simulink model "Panel_Equation"  (R2022b)
settings: Solver=VariableStepAuto  StartTime=0.0  StopTime=10.0  RelTol=1e-3
model workspace (MAT data in the model file):
  J = 8.6
  Kd = 5
settings Model: Creator=adlercohen  LastModifiedBy=adlercohen

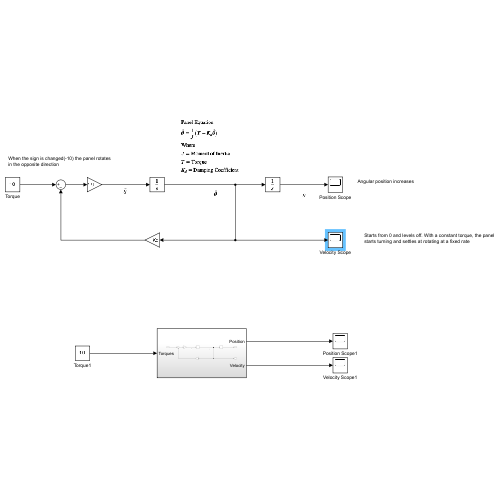
[thumbnail: Simulink's stored preview of the top-level diagram]
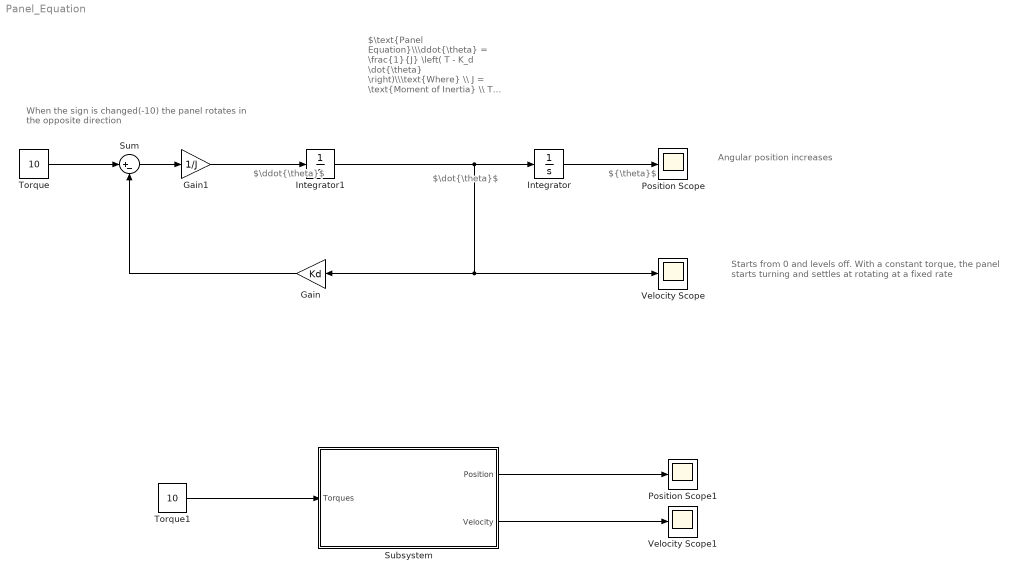
== system Panel_Equation ==
  note: When the sign is changed(-10) the panel rotates
      | in the opposite direction
  note: Starts from 0 and levels off. With a constant torque, the panel
      | starts turning and settles at rotating at a fixed rate
  note: Angular position increases
  note: $\dot{\theta}$
  note: $\text{Panel Equation}\\\ddot{\theta} = \frac{1}{J} \left( T - K_d \dot{\theta} \right)\\\text{Where} \\ J = \text{Moment of Inertia} \\ T = \text{Torque} \\ K_d = \text{Damping Coefficient}$
  note: $\ddot{\theta}$
  note: ${\theta}$
  Gain : Gain  Gain=Kd
  Gain1 : Gain  Gain=1/J
  Integrator : Integrator
  Integrator1 : Integrator
  Position Scope : Scope
  Position Scope1 : Scope
  Subsystem : Subsystem
  Sum : Sum  Inputs=|+-
  Torque : Constant  Value=10
  Torque1 : Constant  Value=10
  Velocity Scope : Scope
  Velocity Scope1 : Scope
  wires:
  Integrator1/1 -> Gain/1, Velocity Scope/1, Integrator/1
  Integrator/1 -> Position Scope/1
  Sum/1 -> Gain1/1
  Torque/1 -> Sum/1
  Gain/1 -> Sum/2
  Gain1/1 -> Integrator1/1
  Torque1/1 -> Subsystem/1(Torques)
  Subsystem/1(Position) -> Position Scope1/1
  Subsystem/2(Velocity) -> Velocity Scope1/1

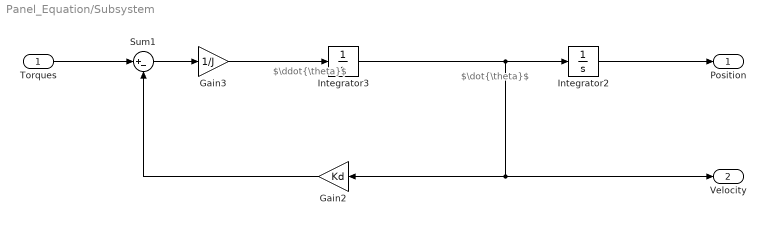
== system Panel_Equation/Subsystem ==
  note: $\ddot{\theta}$
  note: $\dot{\theta}$
  Torques : Inport
  Gain2 : Gain  Gain=Kd
  Gain3 : Gain  Gain=1/J
  Integrator2 : Integrator
  Integrator3 : Integrator
  Sum1 : Sum  Inputs=|+-
  Position : Outport
  Velocity : Outport  Port=2
  wires:
  Torques/1 -> Sum1/1
  Integrator3/1 -> Velocity/1, Gain2/1, Integrator2/1
  Gain2/1 -> Sum1/2
  Sum1/1 -> Gain3/1
  Integrator2/1 -> Position/1
  Gain3/1 -> Integrator3/1
